simulink model "lineaEEC"  (R2015a)
settings: Solver=ode45  StartTime=0.0  StopTime=0.16  RelTol=1e-3
undefined symbols (not defined in the file): Sb, Vbas
libraries: powerlib x74
settings Model: CovSFcnEnable=off  Creator=ricardo  LastModifiedBy=USUARIO
settings DebuggingCC: SolverPrmCheckMsg=warning

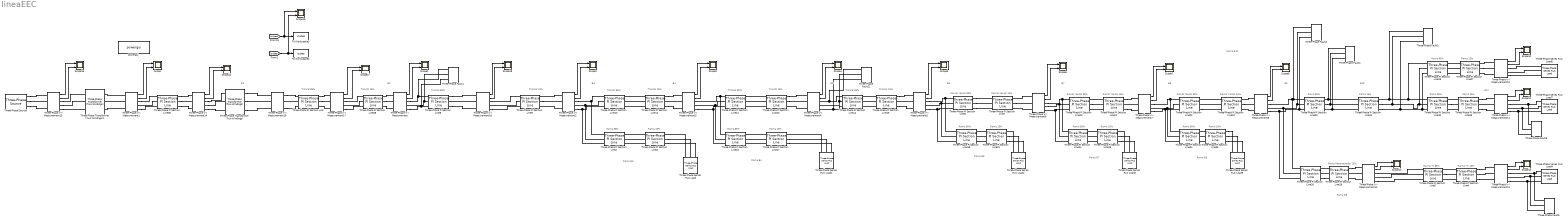
== system lineaEEC ==
  note: B11
  note: B10
  note: B9
  note: B8
  note: B7
  note: B6
  note: B5
  note: B4
  note: Rama B3
  note: B3
  note: B2
  note: B1
  note: Rama 85%
  note: Troncal 85%
  note: Troncal 15%
  note: Rama 15%
  note: Troncal 85%
  note: Troncal 15%
  note: Troncal 85%
  note: Troncal 15%
  note: Troncal 85%
  note: Troncal 15%
  note: Troncal 85%
  note: Troncal 15%
  note: Rama 85%
  note: Rama 15%
  note: Rama 85%
  note: Rama 15%
  note: Ramal Yacopi 85%
  note: Ramal Yacopi 15%
  note: Ramal Yacopi 85%
  note: Ramal Yacopi 15%
  note: Ramal Yacopi 85%
  note: Ramal Yacopi 15%
  note: Rama 85%
  note: Rama 15%
  note: Rama Reconectador 15%
  note: Rama 85%
  note: Rama 15%
  note: Rama 85%
  note: Rama 15%
  note: Ramal 7k 15%
  note: Ramal 7k 85%
  note: Rama 85%
  note: Rama 15%
  note: Rama 85%
  note: Rama 15%
  note: Rama B4
  note: Rama B6
  note: Rama B7
  note: Rama B8
  note: Rama B9
  note: Rama B10
  Scope{,1..8,10..15,17..19} (18 alike) : Scope  NumInputPorts=2
      Scope settings: YMin=-5~-5  YMax=5~5
      Scope1 settings: YMin=-5~-5  YMax=5~5
      Scope10 settings: YMin=-5~-5  YMax=5~5  SaveName=ScopeData10
      Scope11 settings: YMin=-5~-5  YMax=5~5  SaveName=ScopeData11
      Scope12 settings: YMin=-5~-5  YMax=5~5  SaveName=ScopeData12
      Scope13 settings: YMin=-5~-5  YMax=5~5  SaveName=ScopeData13
      Scope14 settings: YMin=-5~-5  YMax=5~5  SaveName=ScopeData14
      Scope15 settings: YMin=-175000~-1  YMax=100000~1.1  SaveName=ScopeData15
      Scope17 settings: YMin=-5~-5  YMax=5~5  SaveName=ScopeData17
      Scope18 settings: YMin=-5~-5  YMax=5~5  SaveName=ScopeData18
      Scope19 settings: TimeRange=0.03177083333333333  YMin=-4000~-5  YMax=4000~5  SaveName=ScopeData19
      Scope2 settings: YMin=-5~-5  YMax=5~5  SaveName=ScopeData2
      Scope3 settings: YMin=-5~-5  YMax=5~5  SaveName=ScopeData3
      Scope4 settings: YMin=-5~-5  YMax=5~5  SaveName=ScopeData4
      Scope5 settings: YMin=-5~-5  YMax=5~5  SaveName=ScopeData5
      Scope6 settings: YMin=-5~-5  YMax=5~5  SaveName=ScopeData6
      Scope7 settings: YMin=-5~-5  YMax=5~5  SaveName=ScopeData7
      Scope8 settings: YMin=-5~-5  YMax=5~5  SaveName=ScopeData8
  Three-Phase PI Section Line : powerlib/Elements/Three-Phase PI Section Line  LConnTagsString=a|b|c  RConnTagsString=A|B|C  Frequency=60  Resistances=[0.4153 0.4148]  Inductances="[0.001327  0.002029]"  Capacitances=[0.1e-12 0.1e-12]  Length=0.224281
  Three-Phase PI Section Line10 : powerlib/Elements/Three-Phase PI Section Line  LConnTagsString=a|b|c  RConnTagsString=A|B|C  Frequency=60  Resistances=[ 0.4153 0.4148]  Inductances="[0.001327  0.002029]"  Capacitances=[0.1e-12 0.1e-12]  Length=2.627724
  Three-Phase PI Section Line11 : powerlib/Elements/Three-Phase PI Section Line  LConnTagsString=a|b|c  RConnTagsString=A|B|C  Frequency=60  Resistances=[0.8315 0.8307]  Inductances=[0.001263 0.002392]  Capacitances=[0.1e-12 0.1e-12]  Length=0.463716
  Three-Phase PI Section Line12 : powerlib/Elements/Three-Phase PI Section Line  LConnTagsString=a|b|c  RConnTagsString=A|B|C  Frequency=60  Resistances=[ 0.4153 0.4148]  Inductances="[0.001327  0.002029]"  Capacitances=[0.1e-12 0.1e-12]  Length=6.782796
  Three-Phase PI Section Line13 : powerlib/Elements/Three-Phase PI Section Line  LConnTagsString=a|b|c  RConnTagsString=A|B|C  Frequency=60  Resistances=[0.8315 0.8307]  Inductances=[0.001263 0.002392]  Capacitances=[0.1e-12 0.1e-12]  Length=1.196964
  Three-Phase PI Section Line14 : powerlib/Elements/Three-Phase PI Section Line  LConnTagsString=a|b|c  RConnTagsString=A|B|C  Frequency=60  Resistances=[ 0.4153 0.4148]  Inductances="[0.001327  0.002029]"  Capacitances=[0.1e-12 0.1e-12]  Length=2.529787
  Three-Phase PI Section Line15 : powerlib/Elements/Three-Phase PI Section Line  LConnTagsString=a|b|c  RConnTagsString=A|B|C  Frequency=60  Resistances=[0.8315 0.8307]  Inductances=[0.001263 0.002392]  Capacitances=[0.1e-12 0.1e-12]  Length=0.446433
  Three-Phase PI Section Line16 : powerlib/Elements/Three-Phase PI Section Line  LConnTagsString=a|b|c  RConnTagsString=A|B|C  Frequency=60  Resistances=[0.8315 0.8307]  Inductances=[0.001096 0.002727]  Capacitances=[0.1e-12 0.1e-12]  Length=6.782796
  Three-Phase PI Section Line17 : powerlib/Elements/Three-Phase PI Section Line  LConnTagsString=a|b|c  RConnTagsString=A|B|C  Frequency=60  Resistances=[0.8315 0.8307]  Inductances=[0.001311 0.002296]  Capacitances=[0.1e-12 0.1e-12]  Length=1.196964
  Three-Phase PI Section Line18 : powerlib/Elements/Three-Phase PI Section Line  LConnTagsString=a|b|c  RConnTagsString=A|B|C  Frequency=60  Resistances=[0.8315 0.8307]  Inductances=[0.001096 0.002727]  Capacitances=[0.1e-12 0.1e-12]  Length=6.82142765
  Three-Phase PI Section Line19 : powerlib/Elements/Three-Phase PI Section Line  LConnTagsString=a|b|c  RConnTagsString=A|B|C  Frequency=60  Resistances=[0.8315 0.8307]  Inductances=[0.001311 0.002296]  Capacitances=[0.1e-12 0.1e-12]  Length=1.203781
  Three-Phase PI Section Line2 : powerlib/Elements/Three-Phase PI Section Line  LConnTagsString=a|b|c  RConnTagsString=A|B|C  Frequency=60  Resistances=[0.8315 0.8307]  Inductances=[0.001096 0.002727]  Capacitances=[0.1e-12 0.1e-12]  Length=6.5409982
  Three-Phase PI Section Line20 : powerlib/Elements/Three-Phase PI Section Line  LConnTagsString=a|b|c  RConnTagsString=A|B|C  Frequency=60  Resistances=[0.416 0.4151]  Inductances=[0.001023 0.002655]  Capacitances=[0.1e-12 0.1e-12]  Length=1.27075
  Three-Phase PI Section Line21 : powerlib/Elements/Three-Phase PI Section Line  LConnTagsString=a|b|c  RConnTagsString=A|B|C  Frequency=60  Resistances=[0.416 0.4151]  Inductances=[0.001239 0.002225]  Capacitances=[0.1e-12 0.1e-12]  Length=0.22425
  Three-Phase PI Section Line22 : powerlib/Elements/Three-Phase PI Section Line  LConnTagsString=a|b|c  RConnTagsString=A|B|C  Frequency=60  Resistances=[0.416 0.4151]  Inductances=[0.001023 0.002655]  Capacitances=[0.1e-12 0.1e-12]  Length=3.753243
  Three-Phase PI Section Line23 : powerlib/Elements/Three-Phase PI Section Line  LConnTagsString=a|b|c  RConnTagsString=A|B|C  Frequency=60  Resistances=[0.416 0.4151]  Inductances=[0.001239 0.002225]  Capacitances=[0.1e-12 0.1e-12]  Length=0.662337
  Three-Phase PI Section Line24 : powerlib/Elements/Three-Phase PI Section Line  LConnTagsString=a|b|c  RConnTagsString=A|B|C  Frequency=60  Resistances=[0.8315 0.8307]  Inductances=[0.001096 0.002727]  Capacitances=[0.1e-12 0.1e-12]  Length=3.3978495
  Three-Phase PI Section Line25 : powerlib/Elements/Three-Phase PI Section Line  LConnTagsString=a|b|c  RConnTagsString=A|B|C  Frequency=60  Resistances=[0.8315 0.8307]  Inductances=[0.001311 0.002296]  Capacitances=[0.1e-12 0.1e-12]  Length=0.22425
  Three-Phase PI Section Line26 : powerlib/Elements/Three-Phase PI Section Line  LConnTagsString=a|b|c  RConnTagsString=A|B|C  Frequency=60  Resistances=[0.8315 0.8307]  Inductances=[0.001096 0.002727]  Capacitances=[0.1e-12 0.1e-12]  Length=6.3333585
  Three-Phase PI Section Line27 : powerlib/Elements/Three-Phase PI Section Line  LConnTagsString=a|b|c  RConnTagsString=A|B|C  Frequency=60  Resistances=[0.8315 0.8307]  Inductances=[0.001311 0.002296]  Capacitances=[0.1e-12 0.1e-12]  Length=1.117652
  Three-Phase PI Section Line28 : powerlib/Elements/Three-Phase PI Section Line  LConnTagsString=a|b|c  RConnTagsString=A|B|C  Frequency=60  Resistances=[0.416 0.4151]  Inductances=[0.001023 0.002655]  Capacitances=[0.1e-12 0.1e-12]  Length=2.818592
  Three-Phase PI Section Line29 : powerlib/Elements/Three-Phase PI Section Line  LConnTagsString=a|b|c  RConnTagsString=A|B|C  Frequency=60  Resistances=[0.416 0.4151]  Inductances=[0.001239 0.002225]  Capacitances=[0.1e-12 0.1e-12]  Length=0.497399
  Three-Phase PI Section Line3 : powerlib/Elements/Three-Phase PI Section Line  LConnTagsString=a|b|c  RConnTagsString=A|B|C  Frequency=60  Resistances=[0.8315 0.8307]  Inductances=[0.001311 0.002296]  Capacitances=[0.1e-12 0.1e-12]  Length=1.154294
  Three-Phase PI Section Line30 : powerlib/Elements/Three-Phase PI Section Line  LConnTagsString=a|b|c  RConnTagsString=A|B|C  Frequency=60  Resistances=[0.416 0.4151]  Inductances=[0.001096 0.002727]  Capacitances=[0.1e-12 0.1e-12]  Length=3.1708145
  Three-Phase PI Section Line31 : powerlib/Elements/Three-Phase PI Section Line  LConnTagsString=a|b|c  RConnTagsString=A|B|C  Frequency=60  Resistances=[0.416 0.4151]  Inductances=[0.001311 0.002296]  Capacitances=[0.1e-12 0.1e-12]  Length=0.559556
  Three-Phase PI Section Line32 : powerlib/Elements/Three-Phase PI Section Line  LConnTagsString=a|b|c  RConnTagsString=A|B|C  Frequency=60  Resistances=[0.416 0.4151]  Inductances=[0.001096 0.002727]  Capacitances=[0.1e-12 0.1e-12]  Length=8.8518235
  Three-Phase PI Section Line33 : powerlib/Elements/Three-Phase PI Section Line  LConnTagsString=a|b|c  RConnTagsString=A|B|C  Frequency=60  Resistances=[0.416 0.4151]  Inductances=[0.001311 0.002296]  Capacitances=[0.1e-12 0.1e-12]  Length=1.562087
  Three-Phase PI Section Line34 : powerlib/Elements/Three-Phase PI Section Line  LConnTagsString=a|b|c  RConnTagsString=A|B|C  Frequency=60  Resistances=[0.8315 0.8307]  Inductances=[0.001096 0.002727]  Capacitances=[0.1e-12 0.1e-12]  Length=4.8514005
  Three-Phase PI Section Line35 : powerlib/Elements/Three-Phase PI Section Line  LConnTagsString=a|b|c  RConnTagsString=A|B|C  Frequency=60  Resistances=[0.8315 0.8307]  Inductances=[0.001311 0.002296]  Capacitances=[0.1e-12 0.1e-12]  Length=0.85613
  Three-Phase PI Section Line36 : powerlib/Elements/Three-Phase PI Section Line  LConnTagsString=a|b|c  RConnTagsString=A|B|C  Frequency=60  Resistances=[ 0.41586 0.82784]  Inductances="[ 1.3743e-3  4.2583e-3]"  Capacitances=[0.00825e-6 0.00588e-6]  Length=9
  Three-Phase PI Section Line38 : powerlib/Elements/Three-Phase PI Section Line  LConnTagsString=a|b|c  RConnTagsString=A|B|C  Frequency=60  Resistances=[0.8315 0.8307]  Inductances=[0.001263 0.002392]  Capacitances=[0.1e-12 0.1e-12]  Length=0.039579
  Three-Phase PI Section Line4 : powerlib/Elements/Three-Phase PI Section Line  LConnTagsString=a|b|c  RConnTagsString=A|B|C  Frequency=60  Resistances=[0.5235 0.5228]  Inductances=[0.001263 0.002248]  Capacitances=[0.1e-12 0.1e-12]  Length=1.05
  Three-Phase PI Section Line5 : powerlib/Elements/Three-Phase PI Section Line  LConnTagsString=a|b|c  RConnTagsString=A|B|C  Frequency=60  Resistances=[0.5238 0.523]  Inductances=[0.001048 0.002679]  Capacitances=[0.1e-12 0.1e-12]  Length=5.95
  Three-Phase PI Section Line6 : powerlib/Elements/Three-Phase PI Section Line  LConnTagsString=a|b|c  RConnTagsString=A|B|C  Frequency=60  Resistances=[0.416 0.4151]  Inductances=[0.001023 0.002655]  Capacitances=[0.1e-12 0.1e-12]  Length=2.9021805
  Three-Phase PI Section Line7 : powerlib/Elements/Three-Phase PI Section Line  LConnTagsString=a|b|c  RConnTagsString=A|B|C  Frequency=60  Resistances=[0.416 0.4151]  Inductances=[0.001239 0.002225]  Capacitances=[0.1e-12 0.1e-12]  Length=0.51215
  Three-Phase PI Section Line8 : powerlib/Elements/Three-Phase PI Section Line  LConnTagsString=a|b|c  RConnTagsString=A|B|C  Frequency=60  Resistances=[0.4153 0.4148]  Inductances="[0.001327  0.002029]"  Capacitances=[0.1e-12 0.1e-12]  Length=8.4235221
  Three-Phase PI Section Line9 : powerlib/Elements/Three-Phase PI Section Line  LConnTagsString=a|b|c  RConnTagsString=A|B|C  Frequency=60  Resistances=[0.8315 0.8307]  Inductances=[0.001263 0.002392]  Capacitances=[0.1e-12 0.1e-12]  Length=1.486504
  Three-Phase Series RLC Load : powerlib/Elements/Three-Phase Series RLC Load  LConnTagsString=A|B|C  Configuration=Y (grounded)  NominalVoltage=Vbas  NominalFrequency=60  ActivePower=7330  InductivePower=2140  CapacitivePower=0  Measurements=Branch voltages and currents  LoadType=constant PQ
  Three-Phase Series RLC Load1 : powerlib/Elements/Three-Phase Series RLC Load  LConnTagsString=A|B|C  Configuration=Y (grounded)  NominalVoltage=Vbas  NominalFrequency=60  ActivePower=16060  InductivePower=4690  CapacitivePower=0  Measurements=Branch voltages and currents  LoadType=constant Z
  Three-Phase Series RLC Load2 : powerlib/Elements/Three-Phase Series RLC Load  LConnTagsString=A|B|C  Configuration=Y (grounded)  NominalVoltage=Vbas  NominalFrequency=60  ActivePower=5120  InductivePower=1490  CapacitivePower=0  Measurements=Branch voltages and currents  LoadType=constant Z
  Three-Phase Series RLC Load3 : powerlib/Elements/Three-Phase Series RLC Load  LConnTagsString=A|B|C  Configuration=Y (grounded)  NominalVoltage=Vbas  NominalFrequency=60  ActivePower=10240  InductivePower=2990  CapacitivePower=0  Measurements=Branch voltages and currents  LoadType=constant Z
  Three-Phase Series RLC Load4 : powerlib/Elements/Three-Phase Series RLC Load  LConnTagsString=A|B|C  Configuration=Y (grounded)  NominalVoltage=Vbas  NominalFrequency=60  ActivePower=9430  InductivePower=2750  CapacitivePower=0  Measurements=Branch voltages and currents  LoadType=constant Z
  Three-Phase Series RLC Load5 : powerlib/Elements/Three-Phase Series RLC Load  LConnTagsString=A|B|C  Configuration=Y (grounded)  NominalVoltage=Vbas  NominalFrequency=60  ActivePower=28640  InductivePower=8350  CapacitivePower=0  Measurements=Branch voltages and currents  LoadType=constant Z
  Three-Phase Series RLC Load6 : powerlib/Elements/Three-Phase Series RLC Load  LConnTagsString=A|B|C  Configuration=Y (grounded)  NominalVoltage=Vbas  NominalFrequency=60  ActivePower=10130  InductivePower=2950  CapacitivePower=0  Measurements=Branch voltages and currents  LoadType=constant Z
  Three-Phase Series RLC Load7 : powerlib/Elements/Three-Phase Series RLC Load  LConnTagsString=A|B|C  Configuration=Y (grounded)  NominalVoltage=Vbas  NominalFrequency=60  ActivePower=6980  InductivePower=2040  CapacitivePower=0  Measurements=Branch voltages and currents  LoadType=constant Z
  Three-Phase Transformer (Two Windings) : powerlib/Elements/Three-Phase Transformer (Two Windings)  Winding1Connection=Yg  Winding2Connection=Yg  CoreType=Three single-phase transformers  SetSaturation=off  Hysteresis=off  DataFile='hysteresis'  SetInitialFlux=off  Measurements=None  UNITS=pu  NominalPower=[Sb , 60 ]  Winding1=[ 34500 , 0 , 0.0273 ]  Winding2=[Vbas , 0 , 0.0273 ]  Rm=500  Lm=500  L0=0.5  Saturation=[ 0,0 ; 0.0024,1.2 ; 1.0,1.52 ]  InitialFluxes=[ 0.8 , -0.8 , 0.7 ]  MoreParameters=off  BreakLoop=off  DataType=off  TransfoNumber=1
  Three-Phase Transformer (Two Windings)1 : powerlib/Elements/Three-Phase Transformer (Two Windings)  Winding1Connection=Yg  Winding2Connection=Yg  CoreType=Three single-phase transformers  SetSaturation=off  Hysteresis=off  DataFile='hysteresis'  SetInitialFlux=off  Measurements=None  UNITS=pu  NominalPower=[ 40e6 , 60 ]  Winding1=[ 115000 , 0 , 0.06 ]  Winding2=[ 34500 , 0 , 0.06 ]  Rm=500  Lm=500  L0=0.5  Saturation=[ 0,0 ; 0.0024,1.2 ; 1.0,1.52 ]  InitialFluxes=[ 0.8 , -0.8 , 0.7 ]  MoreParameters=off  BreakLoop=off  DataType=off  TransfoNumber=1
  Three-Phase V-I Measurement{,1..8,10..15,17..18} (17 alike) : powerlib/Measurements/Three-Phase V-I Measurement  VoltageMeasurement=phase-to-phase  SetLabelV=off  LabelV=Vabc  Vpu=off  VpuLL=off  CurrentMeasurement=yes  SetLabelI=off  LabelI=Iabc  Ipu=off  Pbase=100e6  Vbase=500e3  OutputType=Complex  PhasorSimulation=off  PSBequivalent=0
  Three-Phase V-I Measurement16 : powerlib/Measurements/Three-Phase V-I Measurement  VoltageMeasurement=phase-to-ground  SetLabelV=on  LabelV=Vsubes  Vpu=off  VpuLL=off  CurrentMeasurement=yes  SetLabelI=on  LabelI=Isubes  Ipu=off  Pbase=100e6  Vbase=500e3  OutputType=Complex  PhasorSimulation=off  PSBequivalent=0
  Three-Phase Fault1 : powerlib/Elements/Three-Phase Fault  InitialStates=0  FaultA=off  FaultB=off  FaultC=off  GroundFault=off  SwitchTimes="[3/60  6/60]"  External=off  SwitchStatus=NaN  FaultResistance=0.010  GroundResistance=0.01  SnubberResistance=1e6  SnubberCapacitance=inf  Measurements=None
  Three-Phase Fault2 : powerlib/Elements/Three-Phase Fault  InitialStates=0  FaultA=off  FaultB=off  FaultC=off  GroundFault=off  SwitchTimes="[3/60  6/60]"  External=off  SwitchStatus=NaN  FaultResistance=0.01  GroundResistance=0.01  SnubberResistance=1e6  SnubberCapacitance=inf  Measurements=None
  Three-Phase Fault21 : powerlib/Elements/Three-Phase Fault  InitialStates=0  FaultA=off  FaultB=off  FaultC=off  GroundFault=off  SwitchTimes="[3/60  6/60]"  External=off  SwitchStatus=NaN  FaultResistance=0.001  GroundResistance=0.01  SnubberResistance=1e6  SnubberCapacitance=inf  Measurements=None
  Three-Phase Fault3 : powerlib/Elements/Three-Phase Fault  InitialStates=0  FaultA=off  FaultB=off  FaultC=off  GroundFault=off  SwitchTimes="[3/60  6/60]"  External=off  SwitchStatus=NaN  FaultResistance=20  GroundResistance=0.01  SnubberResistance=1e6  SnubberCapacitance=inf  Measurements=None
  Three-Phase Fault4 : powerlib/Elements/Three-Phase Fault  InitialStates=0  FaultA=off  FaultB=off  FaultC=off  GroundFault=off  SwitchTimes="[3/60  6/60]"  External=off  SwitchStatus=NaN  FaultResistance=0.01  GroundResistance=0.01  SnubberResistance=1e6  SnubberCapacitance=inf  Measurements=None
  Three-Phase Fault5 : powerlib/Elements/Three-Phase Fault  InitialStates=0  FaultA=off  FaultB=off  FaultC=off  GroundFault=off  SwitchTimes="[3/60  6/60]"  External=off  SwitchStatus=NaN  FaultResistance=5  GroundResistance=0.01  SnubberResistance=1e6  SnubberCapacitance=inf  Measurements=None
  Three-Phase Fault6 : powerlib/Elements/Three-Phase Fault  InitialStates=0  FaultA=off  FaultB=off  FaultC=on  GroundFault=on  SwitchTimes="[3/60  6/60]"  External=off  SwitchStatus=NaN  FaultResistance=0.001  GroundResistance=0.01  SnubberResistance=1e6  SnubberCapacitance=inf  Measurements=None
  Three-Phase Source : powerlib/Electrical Sources/Three-Phase Source  Voltage=115000  PhaseAngle=0  Frequency=60  InternalConnection=Yg  SpecifyImpedance=on  Resistance=0.8929  Inductance=16.58e-3  ShortCircuitLevel=100e6  BaseVoltage=115000  XRratio=7  BusType=swing  Pref=0  Qref=0  Qmin=-inf  Qmax=inf
  To Workspace2 : ToWorkspace  VariableName=Isubes  SampleTime=-1
  To Workspace3 : ToWorkspace  VariableName=Vsubes  SampleTime=-1
  powergui : powerlib/powergui  Priority=1  SimulationMode=Discrete  SolverType=Tustin  SampleTime=5.208333e-4  frequency=60  SPID=off  DisableSnubberDevices=off  DisableRonSwitches=off  DisableVfSwitches=off  SwTol=0  DisplayEquations=off  Interpol=off  methode=off  Ts=0  FunctionMessages=off  echomessages=off  HookPort=off  EnableUseOfTLC=off  x0status=blocks  frequencyindice=0  Pbase=100e6  ErrMax=1e-4  Iterations=100  UnitsV=kV  UnitsW=MW  buscounter=0  RestoreLinks=warning  ResistiveCurrentMeasurement=off  Frange=[0:2:500]  Ylog=off  Xlog=on  ShowGrid=off  save=off  variable=ZData  structure=0  ZoomFFT=off  StartTime=0.0  cycles=1  DisplayStyle=1  fundamental=60  FreqAxis=off  MaxFrequency=1000  frequencyindicesteady=1  RmsSteady=1  display=off
  wires:
  Three-Phase V-I Measurement/2 -> Scope1/2
  Three-Phase V-I Measurement/1 -> Scope1/1
  Three-Phase V-I Measurement2/2 -> Scope2/2
  Three-Phase V-I Measurement2/1 -> Scope2/1
  Three-Phase V-I Measurement3/2 -> Scope3/2
  Three-Phase V-I Measurement3/1 -> Scope3/1
  Three-Phase V-I Measurement4/2 -> Scope4/2
  Three-Phase V-I Measurement4/1 -> Scope4/1
  Three-Phase V-I Measurement5/2 -> Scope5/2
  Three-Phase V-I Measurement5/1 -> Scope5/1
  Three-Phase V-I Measurement6/2 -> Scope6/2
  Three-Phase V-I Measurement6/1 -> Scope6/1
  Three-Phase V-I Measurement7/2 -> Scope7/2
  Three-Phase V-I Measurement7/1 -> Scope7/1
  Three-Phase V-I Measurement8/2 -> Scope8/2
  Three-Phase V-I Measurement8/1 -> Scope8/1
  Three-Phase V-I Measurement11/2 -> Scope11/2
  Three-Phase V-I Measurement11/1 -> Scope11/1
  Three-Phase V-I Measurement12/2 -> Scope12/2
  Three-Phase V-I Measurement12/1 -> Scope12/1
  Three-Phase V-I Measurement13/1 -> Scope13/1
  Three-Phase V-I Measurement13/2 -> Scope13/2
  Three-Phase V-I Measurement10/1 -> Scope10/1
  Three-Phase V-I Measurement10/2 -> Scope10/2
  Three-Phase V-I Measurement14/2 -> Scope14/2
  Three-Phase V-I Measurement14/1 -> Scope14/1
  Three-Phase V-I Measurement1/1 -> Scope/1
  Three-Phase V-I Measurement1/2 -> Scope/2
  Three-Phase V-I Measurement15/1 -> Scope15/1
  Three-Phase V-I Measurement15/2 -> Scope15/2
  Three-Phase V-I Measurement17/2 -> Scope17/2
  Three-Phase V-I Measurement17/1 -> Scope17/1
  Three-Phase V-I Measurement18/2 -> Scope18/2
  Three-Phase V-I Measurement18/1 -> Scope18/1
  [Vsubes] -> Scope19/1, To Workspace3/1
  [Isubes] -> Scope19/2, To Workspace2/1
  connections:
  Three-Phase PI Section Line11/LConn2 -- Three-Phase PI Section Line10/RConn2
  Three-Phase PI Section Line11/LConn3 -- Three-Phase PI Section Line10/RConn3
  Three-Phase PI Section Line11/LConn1 -- Three-Phase PI Section Line10/RConn1
  Three-Phase PI Section Line13/LConn2 -- Three-Phase PI Section Line12/RConn2
  Three-Phase PI Section Line13/LConn3 -- Three-Phase PI Section Line12/RConn3
  Three-Phase PI Section Line13/LConn1 -- Three-Phase PI Section Line12/RConn1
  Three-Phase PI Section Line15/LConn2 -- Three-Phase PI Section Line14/RConn2
  Three-Phase PI Section Line15/LConn3 -- Three-Phase PI Section Line14/RConn3
  Three-Phase PI Section Line15/LConn1 -- Three-Phase PI Section Line14/RConn1
  Three-Phase PI Section Line3/LConn1 -- Three-Phase PI Section Line2/RConn1
  Three-Phase PI Section Line3/LConn2 -- Three-Phase PI Section Line2/RConn2
  Three-Phase PI Section Line3/LConn3 -- Three-Phase PI Section Line2/RConn3
  Three-Phase Series RLC Load/LConn1 -- Three-Phase PI Section Line3/RConn1
  Three-Phase PI Section Line3/RConn2 -- Three-Phase Series RLC Load/LConn2
  Three-Phase PI Section Line3/RConn3 -- Three-Phase Series RLC Load/LConn3
  Three-Phase PI Section Line17/LConn2 -- Three-Phase PI Section Line16/RConn2
  Three-Phase Series RLC Load1/LConn1 -- Three-Phase PI Section Line17/RConn1
  Three-Phase PI Section Line17/RConn2 -- Three-Phase Series RLC Load1/LConn2
  Three-Phase PI Section Line17/RConn3 -- Three-Phase Series RLC Load1/LConn3
  Three-Phase PI Section Line17/LConn3 -- Three-Phase PI Section Line16/RConn3
  Three-Phase PI Section Line17/LConn1 -- Three-Phase PI Section Line16/RConn1
  Three-Phase Series RLC Load2/LConn1 -- Three-Phase PI Section Line19/RConn1
  Three-Phase PI Section Line19/LConn3 -- Three-Phase PI Section Line18/RConn3
  Three-Phase PI Section Line19/LConn1 -- Three-Phase PI Section Line18/RConn1
  Three-Phase PI Section Line19/LConn2 -- Three-Phase PI Section Line18/RConn2
  Three-Phase PI Section Line19/RConn2 -- Three-Phase Series RLC Load2/LConn2
  Three-Phase PI Section Line19/RConn3 -- Three-Phase Series RLC Load2/LConn3
  Three-Phase PI Section Line25/LConn2 -- Three-Phase PI Section Line24/RConn2
  Three-Phase PI Section Line25/LConn3 -- Three-Phase PI Section Line24/RConn3
  Three-Phase PI Section Line25/RConn2 -- Three-Phase Series RLC Load3/LConn2
  Three-Phase PI Section Line25/LConn1 -- Three-Phase PI Section Line24/RConn1
  Three-Phase PI Section Line25/RConn3 -- Three-Phase Series RLC Load3/LConn3
  Three-Phase Series RLC Load3/LConn1 -- Three-Phase PI Section Line25/RConn1
  Three-Phase PI Section Line6/RConn1 -- Three-Phase PI Section Line7/LConn1
  Three-Phase PI Section Line6/RConn2 -- Three-Phase PI Section Line7/LConn2
  Three-Phase PI Section Line6/RConn3 -- Three-Phase PI Section Line7/LConn3
  Three-Phase PI Section Line21/LConn1 -- Three-Phase PI Section Line20/RConn1
  Three-Phase PI Section Line20/RConn2 -- Three-Phase PI Section Line21/LConn2
  Three-Phase PI Section Line21/LConn3 -- Three-Phase PI Section Line20/RConn3
  Three-Phase PI Section Line23/LConn1 -- Three-Phase PI Section Line22/RConn1
  Three-Phase PI Section Line23/LConn2 -- Three-Phase PI Section Line22/RConn2
  Three-Phase PI Section Line22/RConn3 -- Three-Phase PI Section Line23/LConn3
  Three-Phase PI Section Line35/RConn1 -- Three-Phase Series RLC Load5/LConn1
  Three-Phase PI Section Line35/RConn2 -- Three-Phase Series RLC Load5/LConn2
  Three-Phase PI Section Line35/RConn3 -- Three-Phase Series RLC Load5/LConn3
  Three-Phase PI Section Line28/RConn3 -- Three-Phase PI Section Line29/LConn3
  Three-Phase PI Section Line29/LConn1 -- Three-Phase PI Section Line28/RConn1
  Three-Phase PI Section Line29/LConn2 -- Three-Phase PI Section Line28/RConn2
  Three-Phase PI Section Line31/LConn1 -- Three-Phase Fault4/LConn1 -- Three-Phase PI Section Line30/RConn1
  Three-Phase PI Section Line30/RConn2 -- Three-Phase Fault4/LConn2 -- Three-Phase PI Section Line31/LConn2
  Three-Phase PI Section Line31/LConn3 -- Three-Phase Fault4/LConn3 -- Three-Phase PI Section Line30/RConn3
  Three-Phase PI Section Line32/RConn2 -- Three-Phase PI Section Line33/LConn2
  Three-Phase PI Section Line33/LConn3 -- Three-Phase PI Section Line32/RConn3
  Three-Phase PI Section Line33/LConn1 -- Three-Phase PI Section Line32/RConn1
  Three-Phase PI Section Line35/LConn3 -- Three-Phase PI Section Line34/RConn3
  Three-Phase PI Section Line35/LConn2 -- Three-Phase PI Section Line34/RConn2
  Three-Phase PI Section Line35/LConn1 -- Three-Phase PI Section Line34/RConn1
  Three-Phase PI Section Line27/LConn2 -- Three-Phase PI Section Line26/RConn2
  Three-Phase PI Section Line27/LConn3 -- Three-Phase PI Section Line26/RConn3
  Three-Phase PI Section Line27/LConn1 -- Three-Phase PI Section Line26/RConn1
  Three-Phase PI Section Line38/RConn1 -- Three-Phase V-I Measurement/LConn1
  Three-Phase PI Section Line38/RConn2 -- Three-Phase V-I Measurement/LConn2
  Three-Phase PI Section Line38/RConn3 -- Three-Phase V-I Measurement/LConn3
  Three-Phase V-I Measurement/RConn1 -- Three-Phase Fault1/LConn1 -- Three-Phase PI Section Line8/LConn1
  Three-Phase PI Section Line8/LConn2 -- Three-Phase Fault1/LConn2 -- Three-Phase V-I Measurement/RConn2
  Three-Phase V-I Measurement/RConn3 -- Three-Phase Fault1/LConn3 -- Three-Phase PI Section Line8/LConn3
  Three-Phase V-I Measurement2/LConn1 -- Three-Phase PI Section Line9/RConn1
  Three-Phase PI Section Line9/RConn2 -- Three-Phase V-I Measurement2/LConn2
  Three-Phase V-I Measurement2/LConn3 -- Three-Phase PI Section Line9/RConn3
  Three-Phase V-I Measurement2/RConn1 -- Three-Phase PI Section Line2/LConn1 -- Three-Phase PI Section Line10/LConn1
  Three-Phase PI Section Line10/LConn2 -- Three-Phase PI Section Line2/LConn2 -- Three-Phase V-I Measurement2/RConn2
  Three-Phase V-I Measurement2/RConn3 -- Three-Phase PI Section Line2/LConn3 -- Three-Phase PI Section Line10/LConn3
  Three-Phase PI Section Line11/RConn1 -- Three-Phase V-I Measurement3/LConn1
  Three-Phase V-I Measurement3/LConn2 -- Three-Phase PI Section Line11/RConn2
  Three-Phase PI Section Line11/RConn3 -- Three-Phase V-I Measurement3/LConn3
  Three-Phase PI Section Line12/LConn1 -- Three-Phase PI Section Line16/LConn1 -- Three-Phase V-I Measurement3/RConn1
  Three-Phase PI Section Line12/LConn2 -- Three-Phase PI Section Line16/LConn2 -- Three-Phase V-I Measurement3/RConn2
  Three-Phase V-I Measurement3/RConn3 -- Three-Phase PI Section Line12/LConn3 -- Three-Phase PI Section Line16/LConn3
  Three-Phase PI Section Line13/RConn1 -- Three-Phase V-I Measurement4/LConn1
  Three-Phase PI Section Line13/RConn2 -- Three-Phase V-I Measurement4/LConn2
  Three-Phase V-I Measurement4/LConn3 -- Three-Phase PI Section Line13/RConn3
  Three-Phase PI Section Line14/LConn1 -- Three-Phase Fault21/LConn1 -- Three-Phase V-I Measurement4/RConn1
  Three-Phase PI Section Line14/LConn2 -- Three-Phase V-I Measurement4/RConn2 -- Three-Phase Fault21/LConn2
  Three-Phase PI Section Line14/LConn3 -- Three-Phase Fault21/LConn3 -- Three-Phase V-I Measurement4/RConn3
  Three-Phase PI Section Line15/RConn1 -- Three-Phase V-I Measurement5/LConn1
  Three-Phase V-I Measurement5/LConn2 -- Three-Phase PI Section Line15/RConn2
  Three-Phase PI Section Line15/RConn3 -- Three-Phase V-I Measurement5/LConn3
  Three-Phase V-I Measurement5/RConn1 -- Three-Phase PI Section Line18/LConn1 -- Three-Phase PI Section Line6/LConn1
  Three-Phase PI Section Line6/LConn2 -- Three-Phase PI Section Line18/LConn2 -- Three-Phase V-I Measurement5/RConn2
  Three-Phase V-I Measurement5/RConn3 -- Three-Phase PI Section Line18/LConn3 -- Three-Phase PI Section Line6/LConn3
  Three-Phase V-I Measurement6/LConn1 -- Three-Phase PI Section Line7/RConn1
  Three-Phase PI Section Line7/RConn2 -- Three-Phase V-I Measurement6/LConn2
  Three-Phase V-I Measurement6/LConn3 -- Three-Phase PI Section Line7/RConn3
  Three-Phase V-I Measurement6/RConn1 -- Three-Phase PI Section Line24/LConn1 -- Three-Phase PI Section Line20/LConn1
  Three-Phase V-I Measurement6/RConn2 -- Three-Phase PI Section Line24/LConn2 -- Three-Phase PI Section Line20/LConn2
  Three-Phase PI Section Line20/LConn3 -- Three-Phase PI Section Line24/LConn3 -- Three-Phase V-I Measurement6/RConn3
  Three-Phase PI Section Line21/RConn1 -- Three-Phase V-I Measurement7/LConn1
  Three-Phase V-I Measurement7/LConn2 -- Three-Phase PI Section Line21/RConn2
  Three-Phase PI Section Line21/RConn3 -- Three-Phase V-I Measurement7/LConn3
  Three-Phase V-I Measurement7/RConn1 -- Three-Phase PI Section Line34/LConn1 -- Three-Phase PI Section Line22/LConn1
  Three-Phase PI Section Line22/LConn2 -- Three-Phase PI Section Line34/LConn2 -- Three-Phase V-I Measurement7/RConn2
  Three-Phase V-I Measurement7/RConn3 -- Three-Phase PI Section Line34/LConn3 -- Three-Phase PI Section Line22/LConn3
  Three-Phase V-I Measurement8/LConn1 -- Three-Phase PI Section Line23/RConn1
  Three-Phase PI Section Line23/RConn2 -- Three-Phase V-I Measurement8/LConn2
  Three-Phase V-I Measurement8/LConn3 -- Three-Phase PI Section Line23/RConn3
  Three-Phase V-I Measurement8/RConn1 -- Three-Phase PI Section Line28/LConn1 -- Three-Phase Fault2/LConn1 -- Three-Phase PI Section Line30/LConn1
  Three-Phase PI Section Line30/LConn2 -- Three-Phase Fault2/LConn2 -- Three-Phase PI Section Line28/LConn2 -- Three-Phase V-I Measurement8/RConn2
  Three-Phase V-I Measurement8/RConn3 -- Three-Phase PI Section Line28/LConn3 -- Three-Phase Fault2/LConn3 -- Three-Phase PI Section Line30/LConn3
  Three-Phase V-I Measurement10/LConn1 -- Three-Phase PI Section Line27/RConn1
  Three-Phase PI Section Line27/RConn2 -- Three-Phase V-I Measurement10/LConn2
  Three-Phase V-I Measurement10/LConn3 -- Three-Phase PI Section Line27/RConn3
  Three-Phase V-I Measurement10/RConn1 -- Three-Phase Series RLC Load6/LConn1
  Three-Phase Series RLC Load6/LConn2 -- Three-Phase V-I Measurement10/RConn2
  Three-Phase V-I Measurement10/RConn3 -- Three-Phase Series RLC Load6/LConn3
  Three-Phase PI Section Line33/RConn1 -- Three-Phase V-I Measurement11/LConn1
  Three-Phase V-I Measurement11/LConn2 -- Three-Phase PI Section Line33/RConn2
  Three-Phase PI Section Line33/RConn3 -- Three-Phase V-I Measurement11/LConn3
  Three-Phase V-I Measurement11/RConn1 -- Three-Phase Fault6/LConn1 -- Three-Phase Series RLC Load7/LConn1
  Three-Phase Series RLC Load7/LConn2 -- Three-Phase Fault6/LConn2 -- Three-Phase V-I Measurement11/RConn2
  Three-Phase V-I Measurement11/RConn3 -- Three-Phase Fault6/LConn3 -- Three-Phase Series RLC Load7/LConn3
  Three-Phase PI Section Line29/RConn1 -- Three-Phase V-I Measurement12/LConn1
  Three-Phase V-I Measurement12/LConn2 -- Three-Phase PI Section Line29/RConn2
  Three-Phase V-I Measurement12/LConn3 -- Three-Phase PI Section Line29/RConn3
  Three-Phase PI Section Line32/LConn1 -- Three-Phase PI Section Line26/LConn1 -- Three-Phase Fault3/LConn1 -- Three-Phase PI Section Line31/RConn1
  Three-Phase PI Section Line31/RConn2 -- Three-Phase Fault3/LConn2 -- Three-Phase PI Section Line26/LConn2 -- Three-Phase PI Section Line32/LConn2
  Three-Phase PI Section Line31/RConn3 -- Three-Phase Fault3/LConn3 -- Three-Phase PI Section Line26/LConn3 -- Three-Phase PI Section Line32/LConn3
  Three-Phase V-I Measurement13/RConn1 -- Three-Phase Fault5/LConn1 -- Three-Phase Series RLC Load4/LConn1
  Three-Phase Series RLC Load4/LConn2 -- Three-Phase Fault5/LConn2 -- Three-Phase V-I Measurement13/RConn2
  Three-Phase V-I Measurement13/RConn3 -- Three-Phase Fault5/LConn3 -- Three-Phase Series RLC Load4/LConn3
  Three-Phase V-I Measurement1/LConn2 -- Three-Phase Transformer (Two Windings)1/RConn2
  Three-Phase V-I Measurement1/LConn1 -- Three-Phase Transformer (Two Windings)1/RConn1
  Three-Phase V-I Measurement1/LConn3 -- Three-Phase Transformer (Two Windings)1/RConn3
  Three-Phase PI Section Line36/RConn3 -- Three-Phase V-I Measurement14/LConn3
  Three-Phase PI Section Line36/RConn2 -- Three-Phase V-I Measurement14/LConn2
  Three-Phase PI Section Line36/RConn1 -- Three-Phase V-I Measurement14/LConn1
  Three-Phase V-I Measurement1/RConn1 -- Three-Phase PI Section Line36/LConn1
  Three-Phase PI Section Line36/LConn2 -- Three-Phase V-I Measurement1/RConn2
  Three-Phase V-I Measurement1/RConn3 -- Three-Phase PI Section Line36/LConn3
  Three-Phase V-I Measurement14/RConn3 -- Three-Phase Transformer (Two Windings)/LConn3
  Three-Phase V-I Measurement14/RConn2 -- Three-Phase Transformer (Two Windings)/LConn2
  Three-Phase V-I Measurement14/RConn1 -- Three-Phase Transformer (Two Windings)/LConn1
  Three-Phase Source/RConn2 -- Three-Phase V-I Measurement15/LConn2
  Three-Phase Source/RConn1 -- Three-Phase V-I Measurement15/LConn1
  Three-Phase Source/RConn3 -- Three-Phase V-I Measurement15/LConn3
  Three-Phase V-I Measurement15/RConn3 -- Three-Phase Transformer (Two Windings)1/LConn3
  Three-Phase V-I Measurement15/RConn2 -- Three-Phase Transformer (Two Windings)1/LConn2
  Three-Phase V-I Measurement15/RConn1 -- Three-Phase Transformer (Two Windings)1/LConn1
  Three-Phase Transformer (Two Windings)/RConn2 -- Three-Phase V-I Measurement16/LConn2
  Three-Phase Transformer (Two Windings)/RConn1 -- Three-Phase V-I Measurement16/LConn1
  Three-Phase Transformer (Two Windings)/RConn3 -- Three-Phase V-I Measurement16/LConn3
  Three-Phase V-I Measurement16/RConn1 -- Three-Phase PI Section Line/LConn1
  Three-Phase PI Section Line/LConn2 -- Three-Phase V-I Measurement16/RConn2
  Three-Phase V-I Measurement16/RConn3 -- Three-Phase PI Section Line/LConn3
  Three-Phase PI Section Line/RConn1 -- Three-Phase V-I Measurement17/LConn1
  Three-Phase PI Section Line/RConn2 -- Three-Phase V-I Measurement17/LConn2
  Three-Phase V-I Measurement17/LConn3 -- Three-Phase PI Section Line/RConn3
  Three-Phase V-I Measurement17/RConn1 -- Three-Phase PI Section Line38/LConn1
  Three-Phase PI Section Line38/LConn2 -- Three-Phase V-I Measurement17/RConn2
  Three-Phase V-I Measurement17/RConn3 -- Three-Phase PI Section Line38/LConn3
  Three-Phase V-I Measurement12/RConn1 -- Three-Phase PI Section Line5/LConn1
  Three-Phase PI Section Line5/LConn2 -- Three-Phase V-I Measurement12/RConn2
  Three-Phase V-I Measurement12/RConn3 -- Three-Phase PI Section Line5/LConn3
  Three-Phase PI Section Line4/LConn1 -- Three-Phase PI Section Line5/RConn1
  Three-Phase PI Section Line5/RConn2 -- Three-Phase PI Section Line4/LConn2
  Three-Phase PI Section Line4/LConn3 -- Three-Phase PI Section Line5/RConn3
  Three-Phase PI Section Line4/RConn1 -- Three-Phase V-I Measurement13/LConn1
  Three-Phase V-I Measurement13/LConn2 -- Three-Phase PI Section Line4/RConn2
  Three-Phase PI Section Line4/RConn3 -- Three-Phase V-I Measurement13/LConn3
  Three-Phase PI Section Line8/RConn1 -- Three-Phase V-I Measurement18/LConn1
  Three-Phase V-I Measurement18/LConn2 -- Three-Phase PI Section Line8/RConn2
  Three-Phase PI Section Line8/RConn3 -- Three-Phase V-I Measurement18/LConn3
  Three-Phase V-I Measurement18/RConn1 -- Three-Phase PI Section Line9/LConn1
  Three-Phase PI Section Line9/LConn2 -- Three-Phase V-I Measurement18/RConn2
  Three-Phase V-I Measurement18/RConn3 -- Three-Phase PI Section Line9/LConn3
